simulink model "Quadrotor_Model_2"  (R2024a)
settings: Solver=ode45  StartTime=0.0  StopTime=350  RelTol=1e-3  EnableMultiTasking=on
values from neighbouring files (symbols this model uses):
  b = 0.07    [project_launch.m]
  g = 9.81    [project_launch.m]
  Jr = 0.0001    [project_launch.m]
  k = 0.09    [project_launch.m]
  L = 0.25    [project_launch.m]
  m = 2.0    (= 2)    [project_launch.m]
settings Model: Creator=boyan  LastModifiedBy=consibic
settings SolverCC: MaxConsecutiveMinStep=2  AlgebraicLoopSolver=TrustRegion
settings DataIOCC: LimitDataPoints=on  SaveFormat=Array  ReturnWorkspaceOutputs=off
settings OptimizationCC: LifeSpan=inf
settings DebuggingCC: SolverPrmCheckMsg=warning  UnconnectedInputMsg=warning  UnconnectedOutputMsg=warning  UnconnectedLineMsg=warning  SFUnexpectedBacktrackingDiag=warning  SFNoUnconditionalDefaultTransitionDiag=warning  SFExecutionAtInitializationDiag=none  ArithmeticOperatorsInVariantConditions=warning
settings HardwareCC: ProdBitPerPointer=32  ProdBitPerSizeT=32  ProdBitPerPtrDiffT=32  ProdLargestAtomicFloat=None  ProdIntDivRoundTo=Undefined  ProdEndianess=Unspecified  ProdWordSize=32  ProdHWDeviceType=32-bit Generic
settings ModelReferenceCC: EnableRefExpFcnMdlSchedulingChecks=on  PropagateSignalLabelsOutOfModel=off
settings SFSimCC: SimUseLocalCustomCode=off  CustomCodeUndefinedFunction=UseInterfaceOnly
settings RTWCC: RTWUseLocalCustomCode=off  GPUComputeCapability=3.5  DLArmComputeVersion=19.05
settings CodeAppCC: StateflowObjectComments=on
settings GRTTargetCC: TargetLangStandard=C89/C90 (ANSI)
settings ConfigComp: CovMetricSettings=dw  CovSaveCumulativeToWorkspaceVar=on  CovSaveSingleToWorkspaceVar=on  CovExternalEMLEnable=off  CovSFcnEnable=off

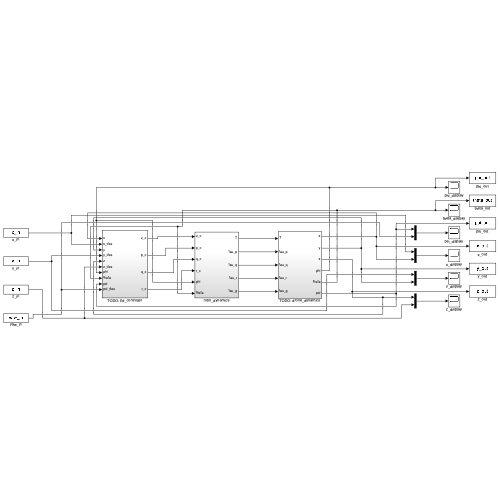
[thumbnail: Simulink's stored preview of the top-level diagram]
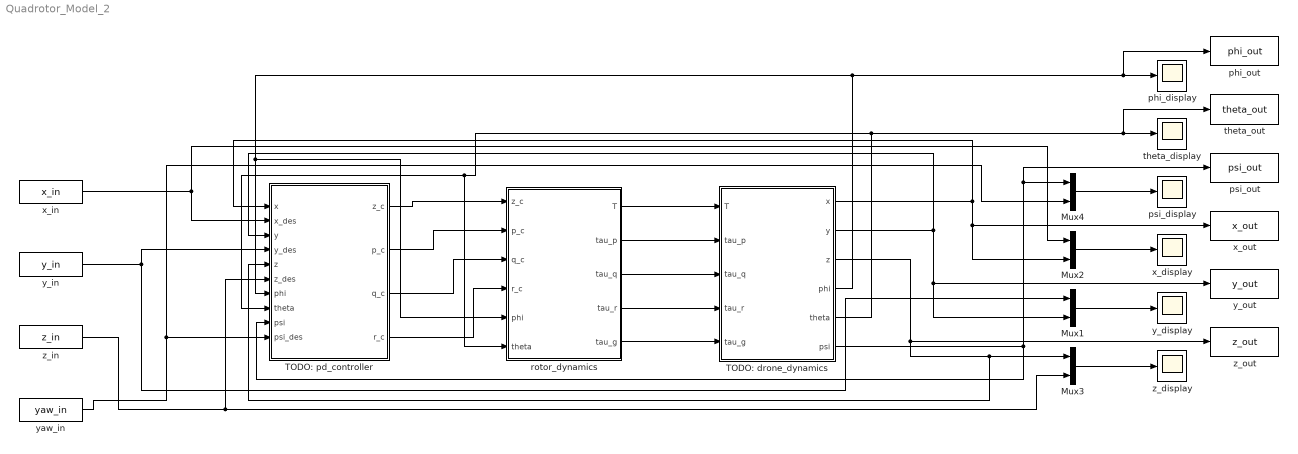
== system Quadrotor_Model_2 ==
  Mux{1..4} (4 alike) : Mux  Inputs=2
  TODO: drone_dynamics : Subsystem
  TODO: pd_controller : Subsystem
  phi_display : Scope
  phi_out : ToWorkspace  VariableName=phi_out  SaveFormat=Timeseries  SampleTime=-1
  psi_display : Scope
  psi_out : ToWorkspace  VariableName=psi_out  SaveFormat=Timeseries  SampleTime=-1
  rotor_dynamics : Subsystem
  theta_display : Scope
  theta_out : ToWorkspace  VariableName=theta_out  SaveFormat=Timeseries  SampleTime=-1
  x_display : Scope
  x_in : FromWorkspace  VariableName=x_in
  x_out : ToWorkspace  VariableName=x_out  SaveFormat=Timeseries  SampleTime=-1
  y_display : Scope
  y_in : FromWorkspace  VariableName=y_in
  y_out : ToWorkspace  VariableName=y_out  SaveFormat=Timeseries  SampleTime=-1
  yaw_in : FromWorkspace  VariableName=yaw_in
  z_display : Scope
  z_in : FromWorkspace  VariableName=z_in
  z_out : ToWorkspace  VariableName=z_out  SaveFormat=Timeseries  SampleTime=-1
  wires:
  rotor_dynamics/1(T) -> TODO: drone_dynamics/1(T)
  rotor_dynamics/2(tau_p) -> TODO: drone_dynamics/2(tau_p)
  TODO: pd_controller/1(z_c) -> rotor_dynamics/1(z_c)
  TODO: pd_controller/2(p_c) -> rotor_dynamics/2(p_c)
  z_in/1 -> TODO: pd_controller/6(z_des), Mux3/2
  Mux1/1 -> y_display/1
  Mux2/1 -> x_display/1
  Mux4/1 -> psi_display/1
  Mux3/1 -> z_display/1
  TODO: drone_dynamics/6(psi) -> TODO: pd_controller/9(psi), psi_out/1, Mux4/1
  y_in/1 -> TODO: pd_controller/4(y_des), Mux1/1
  x_in/1 -> TODO: pd_controller/2(x_des), Mux2/1
  TODO: drone_dynamics/3(z) -> z_out/1, TODO: pd_controller/5(z), Mux3/1
  TODO: drone_dynamics/5(theta) -> theta_out/1, theta_display/1, rotor_dynamics/6(theta), TODO: pd_controller/8(theta)
  TODO: drone_dynamics/2(y) -> TODO: pd_controller/3(y), Mux1/2, y_out/1
  TODO: drone_dynamics/4(phi) -> phi_out/1, phi_display/1, rotor_dynamics/5(phi), TODO: pd_controller/7(phi)
  TODO: drone_dynamics/1(x) -> TODO: pd_controller/1(x), Mux2/2, x_out/1
  rotor_dynamics/5(tau_g) -> TODO: drone_dynamics/5(tau_g)
  rotor_dynamics/3(tau_q) -> TODO: drone_dynamics/3(tau_q)
  rotor_dynamics/4(tau_r) -> TODO: drone_dynamics/4(tau_r)
  yaw_in/1 -> TODO: pd_controller/10(psi_des), Mux4/2
  TODO: pd_controller/4(r_c) -> rotor_dynamics/4(r_c)
  TODO: pd_controller/3(q_c) -> rotor_dynamics/3(q_c)

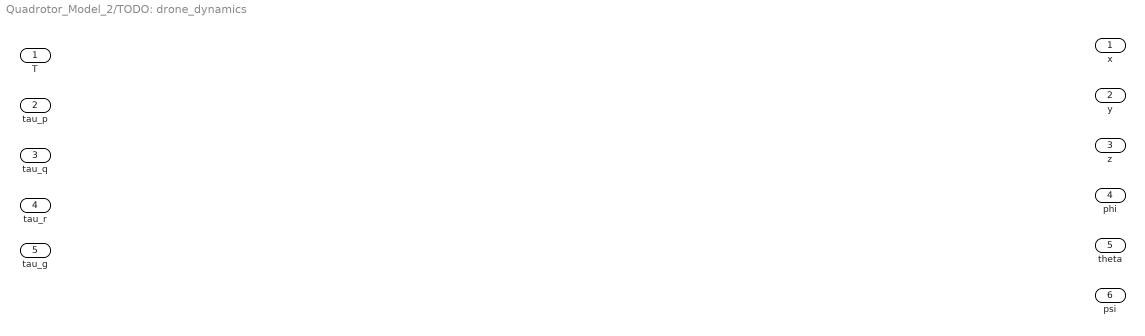
== system Quadrotor_Model_2/TODO: drone_dynamics ==
  T : Inport
  tau_p : Inport  Port=2
  tau_q : Inport  Port=3
  tau_r : Inport  Port=4
  tau_g : Inport  Port=5
  x : Outport
  y : Outport  Port=2
  z : Outport  Port=3
  phi : Outport  Port=4
  theta : Outport  Port=5
  psi : Outport  Port=6

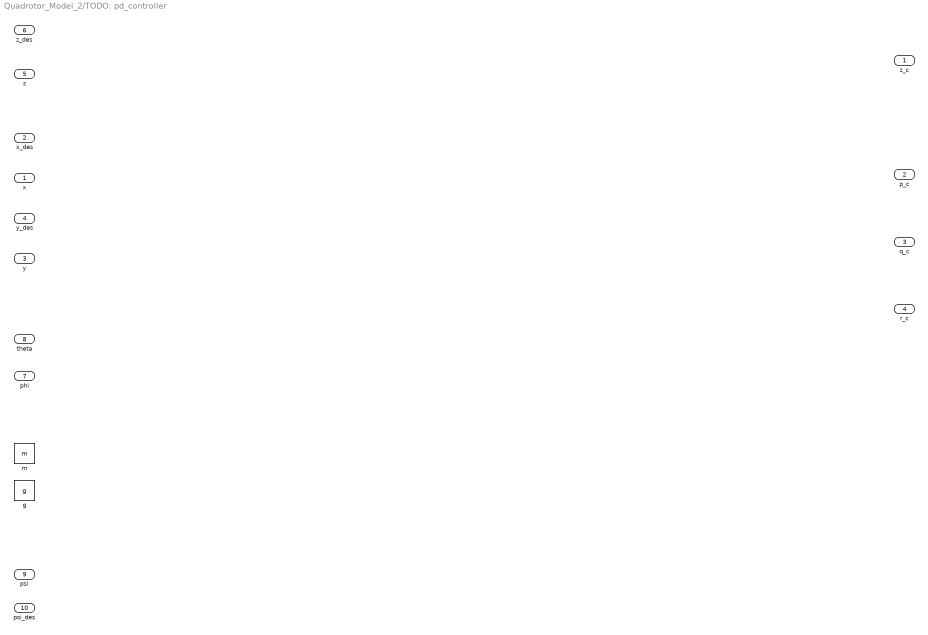
== system Quadrotor_Model_2/TODO: pd_controller ==
  x : Inport
  x_des : Inport  Port=2
  y : Inport  Port=3
  y_des : Inport  Port=4
  z : Inport  Port=5
  z_des : Inport  Port=6
  phi : Inport  Port=7
  theta : Inport  Port=8
  psi : Inport  Port=9
  psi_des : Inport  Port=10
  g : Constant  Value=g
  m : Constant  Value=m
  z_c : Outport
  p_c : Outport  Port=2
  q_c : Outport  Port=3
  r_c : Outport  Port=4

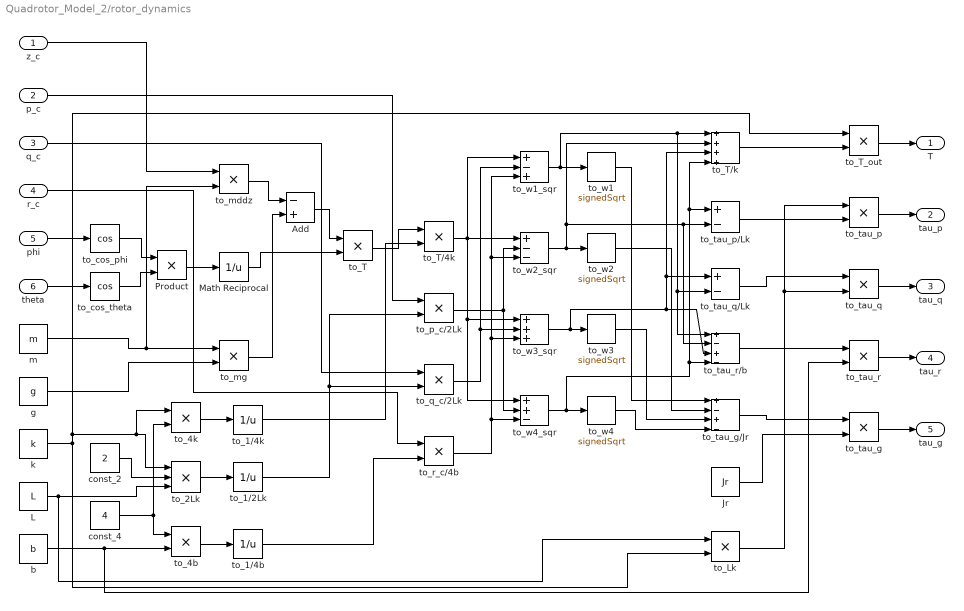
== system Quadrotor_Model_2/rotor_dynamics ==
  z_c : Inport
  p_c : Inport  Port=2
  q_c : Inport  Port=3
  r_c : Inport  Port=4
  phi : Inport  Port=5
  theta : Inport  Port=6
  Add : Sum  Inputs=-+
  Jr : Constant  Value=Jr
  L : Constant  Value=L
  Math Reciprocal : Math  Operator=reciprocal  SignedPower=on
  Product : Product
  b : Constant  Value=b
  const_2 : Constant  Value=2
  const_4 : Constant  Value=4
  g : Constant  Value=g
  k : Constant  Value=k
  m : Constant  Value=m
  to_1/2Lk : Math  Operator=reciprocal  SignedPower=on
  to_1/4b : Math  Operator=reciprocal  SignedPower=on
  to_1/4k : Math  Operator=reciprocal  SignedPower=on
  to_2Lk : Product  Inputs=3
  to_4b : Product
  to_4k : Product
  to_Lk : Product
  to_T : Product
  to_T/4k : Product
  to_T/k : Sum  Inputs=++++
  to_T_out : Product
  to_cos_phi : Trigonometry  Operator=cos
  to_cos_theta : Trigonometry  Operator=cos
  to_mddz : Product
  to_mg : Product
  to_p_c/2Lk : Product
  to_q_c/2Lk : Product
  to_r_c/4b : Product
  to_tau_g : Product
  to_tau_g/Jr : Sum  Inputs=+-+-
  to_tau_p : Product
  to_tau_p/Lk : Sum  Inputs=+-
  to_tau_q : Product
  to_tau_q/Lk : Sum  Inputs=+-
  to_tau_r : Product
  to_tau_r/b : Sum  Inputs=+-+-
  to_w{1..4} (4 alike) : Sqrt  Operator=signedSqrt
  to_w1_sqr : Sum  Inputs=+-+
  to_w2_sqr : Sum  Inputs=+--
  to_w3_sqr : Sum  Inputs=+++
  to_w4_sqr : Sum  Inputs=++-
  T : Outport
  tau_p : Outport  Port=2
  tau_q : Outport  Port=3
  tau_r : Outport  Port=4
  tau_g : Outport  Port=5
  wires:
  phi/1 -> to_cos_phi/1
  theta/1 -> to_cos_theta/1
  to_cos_phi/1 -> Product/1
  to_cos_theta/1 -> Product/2
  Product/1 -> Math Reciprocal/1
  m/1 -> to_mddz/2, to_mg/1
  g/1 -> to_mg/2
  to_mg/1 -> Add/2
  Math Reciprocal/1 -> to_T/2
  Add/1 -> to_T/1
  k/1 -> to_2Lk/1, to_4k/1, to_T_out/1, to_Lk/2
  const_4/1 -> to_4b/1, to_4k/2
  const_2/1 -> to_2Lk/2
  L/1 -> to_2Lk/3, to_Lk/1
  b/1 -> to_tau_r/2, to_4b/2
  to_4k/1 -> to_1/4k/1
  to_2Lk/1 -> to_1/2Lk/1
  to_4b/1 -> to_1/4b/1
  to_T/1 -> to_T/4k/1
  to_1/4k/1 -> to_T/4k/2
  p_c/1 -> to_p_c/2Lk/1
  to_1/2Lk/1 -> to_q_c/2Lk/2, to_p_c/2Lk/2
  q_c/1 -> to_q_c/2Lk/1
  to_1/4b/1 -> to_r_c/4b/2
  r_c/1 -> to_r_c/4b/1
  to_T/4k/1 -> to_w2_sqr/1, to_w3_sqr/1, to_w4_sqr/1, to_w1_sqr/1
  to_q_c/2Lk/1 -> to_w3_sqr/2, to_w1_sqr/2
  to_r_c/4b/1 -> to_w4_sqr/3, to_w3_sqr/3, to_w2_sqr/3, to_w1_sqr/3
  to_p_c/2Lk/1 -> to_w2_sqr/2, to_w4_sqr/2
  to_w1_sqr/1 -> to_w1/1, to_tau_r/b/1, to_tau_q/Lk/2, to_T/k/1
  to_w2_sqr/1 -> to_w2/1, to_tau_r/b/2, to_tau_p/Lk/2, to_T/k/2
  to_w3_sqr/1 -> to_w3/1, to_tau_q/Lk/1, to_T/k/3, to_tau_r/b/3
  to_w4_sqr/1 -> to_w4/1, to_tau_p/Lk/1, to_T/k/4, to_tau_r/b/4
  to_w2/1 -> to_tau_g/Jr/2
  to_w1/1 -> to_tau_g/Jr/1
  to_w3/1 -> to_tau_g/Jr/3
  to_w4/1 -> to_tau_g/Jr/4
  to_T_out/1 -> T/1
  to_T/k/1 -> to_T_out/2
  to_tau_p/1 -> tau_p/1
  to_tau_p/Lk/1 -> to_tau_p/2
  to_tau_q/1 -> tau_q/1
  to_tau_r/1 -> tau_r/1
  to_tau_r/b/1 -> to_tau_r/1
  to_tau_q/Lk/1 -> to_tau_q/1
  to_tau_g/1 -> tau_g/1
  to_tau_g/Jr/1 -> to_tau_g/1
  to_Lk/1 -> to_tau_p/1, to_tau_q/2
  Jr/1 -> to_tau_g/2
  z_c/1 -> to_mddz/1
  to_mddz/1 -> Add/1
